simulink model "hw2_1"  (R2021a)
settings: Solver=VariableStepAuto  StartTime=0.0  StopTime=20  RelTol=1e-3
values from neighbouring files (symbols this model uses):
  B = accelTime/pi    [sineProfile.m]
libraries: raspberrypiBasiclib x2, simulink x1
settings Model: Creator=ku347  LastModifiedBy=ku347

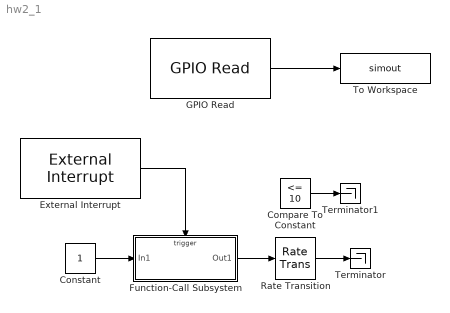
== system hw2_1 ==
  Compare To Constant : simulink/Logic and Bit Operations/Compare To Constant  relop=<=  const=10  OutDataTypeStr=boolean
  Constant : Constant
  External Interrupt : raspberrypiBasiclib/External Interrupt  Board=Pi 4 Model B  Pin=9  PullUp=Pull-down  Mode=Rising  InterruptSimulationInput=off  blockPlatform=Raspberry Pi
      settings: SourceProductBaseCode=RASPPI
  Function-Call Subsystem : Subsystem  TreatAsAtomicUnit=on
  GPIO Read : raspberrypiBasiclib/GPIO Read  board=Model B+  gpio=17  internalResistor=Off  sampleTime=0.1  direction=Input  blockPlatform=Raspberry Pi
      settings: SourceProductBaseCode=RASPPI
  Rate Transition : RateTransition  Deterministic=off
  Terminator : Terminator
  Terminator1 : Terminator
  To Workspace : ToWorkspace  VariableName=simout  SaveFormat=Timeseries  SampleTime=-1
  wires:
  Function-Call Subsystem/1(Out1) -> Rate Transition/1
  Constant/1 -> Function-Call Subsystem/1(In1)
  Rate Transition/1 -> Terminator/1
  External Interrupt/1 -> Function-Call Subsystem/Trigger
  GPIO Read/1 -> To Workspace/1
  Compare To Constant/1 -> Terminator1/1

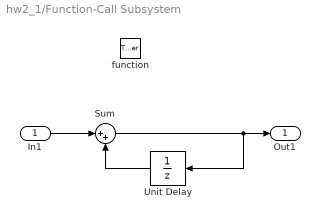
== system hw2_1/Function-Call Subsystem ==
  In1 : Inport
  function : TriggerPort  TriggerType=function-call  VariantControl=(inherit)
  Sum : Sum  Inputs=|++
  Unit Delay : UnitDelay  SampleTime=-1  HasFrameUpgradeWarning=on
  Out1 : Outport
  wires:
  In1/1 -> Sum/1
  Sum/1 -> Unit Delay/1, Out1/1
  Unit Delay/1 -> Sum/2
